simulink model "model2"  (Simulink 7.3)
settings: Solver=ode45  StartTime=0.0  StopTime=10.0  RelTol=1e-3
libraries: simulink x3
settings Model: Creator=IEUser  LastModifiedBy=IEUser

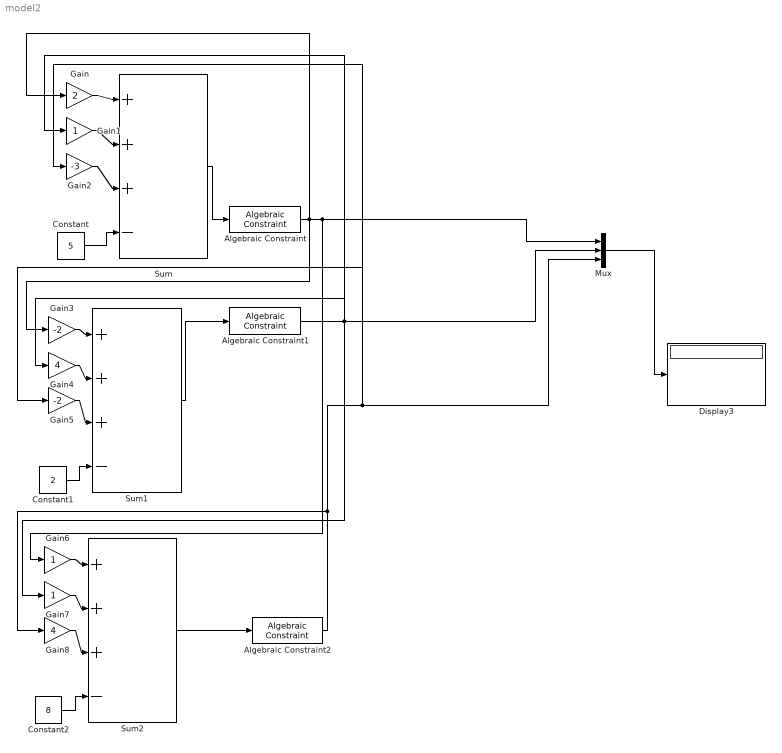
== system model2 ==
  Algebraic Constraint : simulink/Math Operations/Algebraic Constraint  SystemSampleTime=-1  z0=0
  Algebraic Constraint1 : simulink/Math Operations/Algebraic Constraint  SystemSampleTime=-1  z0=0
  Algebraic Constraint2 : simulink/Math Operations/Algebraic Constraint  SystemSampleTime=-1  z0=0
  Constant : Constant  Value=5  OutDataType=fixdt(1, 16)  OutScaling=2^0
  Constant1 : Constant  Value=2  OutDataType=fixdt(1, 16)  OutScaling=2^0
  Constant2 : Constant  Value=8  OutDataType=fixdt(1, 16)  OutScaling=2^0
  Display3 : Display
  Gain : Gain  Gain=2  ParameterDataType=fixdt(1, 16)  ParameterScaling=2^0  OutDataType=fixdt(1, 16)  OutScaling=2^0
  Gain1 : Gain  ParameterDataType=fixdt(1, 16)  ParameterScaling=2^0  OutDataType=fixdt(1, 16)  OutScaling=2^0
  Gain2 : Gain  Gain=-3  ParameterDataType=fixdt(1, 16)  ParameterScaling=2^0  OutDataType=fixdt(1, 16)  OutScaling=2^0
  Gain3 : Gain  Gain=-2  ParameterDataType=fixdt(1, 16)  ParameterScaling=2^0  OutDataType=fixdt(1, 16)  OutScaling=2^0
  Gain4 : Gain  Gain=4  ParameterDataType=fixdt(1, 16)  ParameterScaling=2^0  OutDataType=fixdt(1, 16)  OutScaling=2^0
  Gain5 : Gain  Gain=-2  ParameterDataType=fixdt(1, 16)  ParameterScaling=2^0  OutDataType=fixdt(1, 16)  OutScaling=2^0
  Gain6 : Gain  ParameterDataType=fixdt(1, 16)  ParameterScaling=2^0  OutDataType=fixdt(1, 16)  OutScaling=2^0
  Gain7 : Gain  ParameterDataType=fixdt(1, 16)  ParameterScaling=2^0  OutDataType=fixdt(1, 16)  OutScaling=2^0
  Gain8 : Gain  Gain=4  ParameterDataType=fixdt(1, 16)  ParameterScaling=2^0  OutDataType=fixdt(1, 16)  OutScaling=2^0
  Mux : Mux  Inputs=3
  Sum : Sum  Inputs=+++|-  OutDataType=fixdt(1, 16)  OutScaling=2^0
  Sum1 : Sum  Inputs=+++|-  OutDataType=fixdt(1, 16)  OutScaling=2^0
  Sum2 : Sum  Inputs=+++|-  OutDataType=fixdt(1, 16)  OutScaling=2^0
  wires:
  Algebraic Constraint/1 -> Gain/1, Gain3/1, Mux/1, Gain6/1
  Algebraic Constraint1/1 -> Gain1/1, Gain4/1, Mux/2, Gain7/1
  Algebraic Constraint2/1 -> Gain2/1, Gain5/1, Mux/3, Gain8/1
  Constant/1 -> Sum/4
  Sum/1 -> Algebraic Constraint/1
  Gain1/1 -> Sum/2
  Gain2/1 -> Sum/3
  Constant1/1 -> Sum1/4
  Sum1/1 -> Algebraic Constraint1/1
  Gain3/1 -> Sum1/1
  Gain4/1 -> Sum1/2
  Gain5/1 -> Sum1/3
  Mux/1 -> Display3/1
  Gain/1 -> Sum/1
  Constant2/1 -> Sum2/4
  Sum2/1 -> Algebraic Constraint2/1
  Gain6/1 -> Sum2/1
  Gain7/1 -> Sum2/2
  Gain8/1 -> Sum2/3
